simulink model "Pilot_Joystick_Test"  (R2022b)
settings: Solver=VariableStepAuto  StartTime=0.0  StopTime=100  RelTol=1e-3
libraries: simulink_extras x3, aerolibanimutils x2
settings Model: Creator=PC  LastModifiedBy=PC

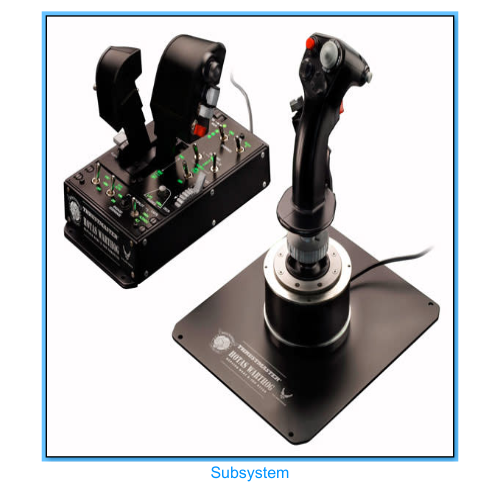
[thumbnail: Simulink's stored preview of the top-level diagram]
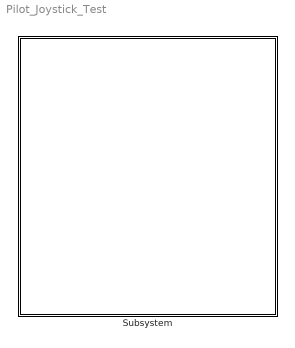
== system Pilot_Joystick_Test ==
  Subsystem : Subsystem
      mask Display: image('Incepter.png'); % Use "Edit Image" on toolstrip to change.

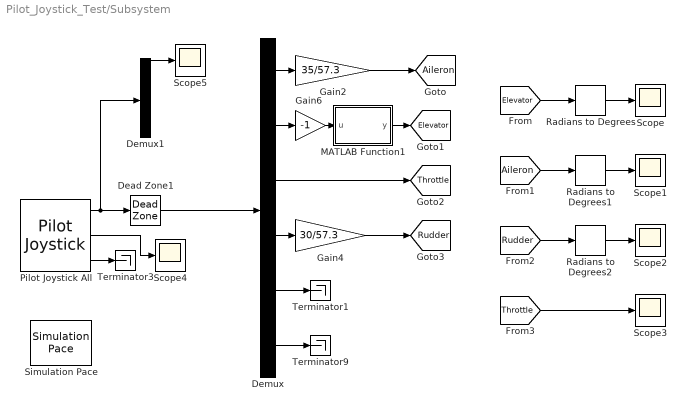
== system Pilot_Joystick_Test/Subsystem ==
  Dead Zone1 : DeadZone  LowerValue=-0.05  UpperValue=0.05
  Demux : Demux  Outputs=6
  Demux1 : Demux  Outputs=6
  Gain2 : Gain  Gain=35/57.3
  Gain4 : Gain  Gain=30/57.3
  Gain6 : Gain  Gain=-1
  MATLAB Function1 : MATLAB Function  TreatAsAtomicUnit=on
  Pilot Joystick All : aerolibanimutils/Pilot Joystick  JoystickID=Joystick1  OutputConfiguration=AllOutputs  SampleTime=1/30
  Radians to Degrees : simulink_extras/Transformations/Radians to Degrees
  Radians to Degrees1 : simulink_extras/Transformations/Radians to Degrees
  Radians to Degrees2 : simulink_extras/Transformations/Radians to Degrees
  Scope{,1..5} (6 alike) : Scope
  Simulation Pace : aerolibanimutils/Simulation Pace  SimulationPace=1  SleepMode=Auto  OutputPaceError=off  SampleTime=1/30
  Terminator1 : Terminator
  Terminator3 : Terminator
  Terminator9 : Terminator
  tag scope: Aileron=global, Elevator=global, Rudder=global, Throttle=global
  wires:
  Demux/3 -> [Throttle]
  Gain2/1 -> [Aileron]
  Demux/5 -> Terminator1/1
  Pilot Joystick All/1 -> Demux1/1, Dead Zone1/1
  Demux/6 -> Terminator9/1
  Gain4/1 -> [Rudder]
  MATLAB Function1/1(y) -> [Elevator]
  Gain6/1 -> MATLAB Function1/1(u)
  Demux/1 -> Gain2/1
  Demux/2 -> Gain6/1
  Dead Zone1/1 -> Demux/1
  Demux/4 -> Gain4/1
  [Elevator] -> Radians to Degrees/1
  [Aileron] -> Radians to Degrees1/1
  [Rudder] -> Radians to Degrees2/1
  [Throttle] -> Scope3/1
  Pilot Joystick All/2 -> Scope4/1
  Pilot Joystick All/3 -> Terminator3/1
  Radians to Degrees/1 -> Scope/1
  Radians to Degrees1/1 -> Scope1/1
  Radians to Degrees2/1 -> Scope2/1
  Demux1/1 -> Scope5/1

== matlab function Pilot_Joystick_Test/Subsystem/MATLAB Function1 ==
  data: u input; y output
function y = fcn(u)
y=(-7.5*u*u+17.5*u)/57.3;
